simulink subsystem "Polynomial_Value"  (R2022b)
settings: Solver=VariableStepAuto  StartTime=0.0  StopTime=10.0  RelTol=1e-3
settings Model: Creator=User  LastModifiedBy=User

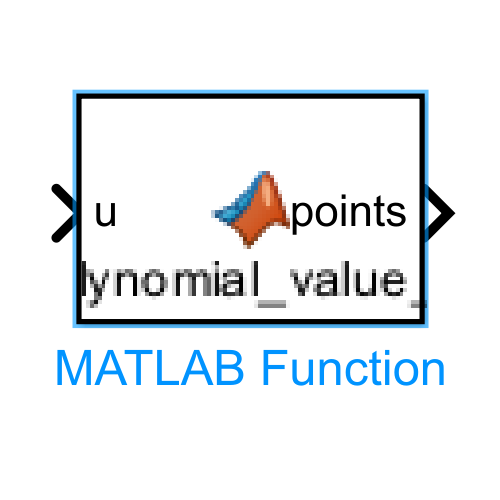
[thumbnail: Simulink's stored preview of the top-level diagram]
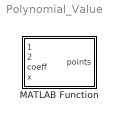
== system Polynomial_Value ==
  MATLAB Function : MATLAB Function  TreatAsAtomicUnit=on

== matlab function Polynomial_Value/MATLAB Function ==
  data: num_degree input; points output; num_point input; coeff input; x input
function points = polynomial_value_m(num_degree, num_point, coeff, x)
    points = polynomial_value(num_degree, num_point, coeff, x);
    
end
